simulink model "third"  (Simulink 7.2)
settings: Solver=ode15s  StartTime=0.0  StopTime=.6  RelTol=1e-3
libraries: powerlib x22, powerlib_extras x13
settings Model: Creator=User  LastModifiedBy=hamed
settings DataIOCC: SaveFormat=StructureWithTime

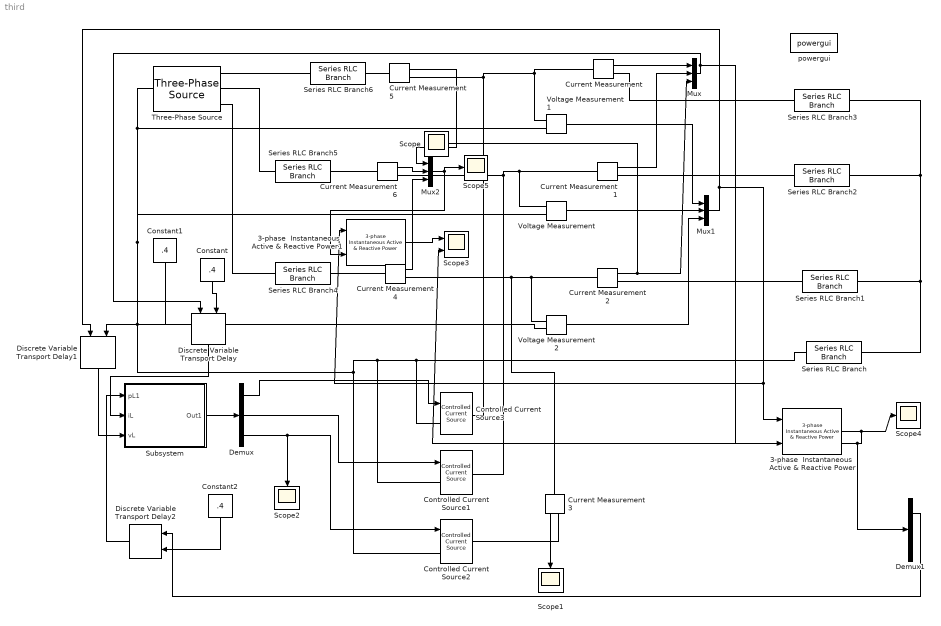
== system third ==
  3-phase  Instantaneous  Active & Reactive Power : powerlib_extras/Measurements/3-phase  Instantaneous  Active & Reactive Power  DialogController=POWERSYS.PowerSysDialog  SystemSampleTime=-1
  3-phase  Instantaneous  Active & Reactive Power1 : powerlib_extras/Measurements/3-phase  Instantaneous  Active & Reactive Power  DialogController=POWERSYS.PowerSysDialog  SystemSampleTime=-1
  Constant : Constant  Orientation=down  Value=.4  OutDataType=sfix(16)  OutScaling=2^0
  Constant1 : Constant  Orientation=down  Value=.4  OutDataType=sfix(16)  OutScaling=2^0
  Constant2 : Constant  Orientation=down  Value=.4  OutDataType=sfix(16)  OutScaling=2^0
  Controlled Current Source1 : powerlib/Electrical Sources/Controlled Current Source  DialogController=POWERSYS.PowerSysDialog  SystemSampleTime=-1  Initialize=on  Source_Type=AC  Amplitude=0  Phase=0  Frequency=0  Measurements=None
  Controlled Current Source2 : powerlib/Electrical Sources/Controlled Current Source  DialogController=POWERSYS.PowerSysDialog  SystemSampleTime=-1  Initialize=on  Source_Type=AC  Amplitude=0  Phase=0  Frequency=0  Measurements=None
  Controlled Current Source3 : powerlib/Electrical Sources/Controlled Current Source  DialogController=POWERSYS.PowerSysDialog  SystemSampleTime=-1  Initialize=on  Source_Type=AC  Amplitude=0  Phase=0  Frequency=0  Measurements=None
  Current Measurement{,1..2,4..6} (6 alike) : powerlib/Measurements/Current Measurement  DialogController=POWERSYS.PowerSysDialog  SystemSampleTime=-1  PhasorSimulation=off  OutputType=Complex  PSBequivalent=0
  Current Measurement3 : powerlib/Measurements/Current Measurement  Orientation=down  DialogController=POWERSYS.PowerSysDialog  SystemSampleTime=-1  PhasorSimulation=off  OutputType=Complex  PSBequivalent=0
  Demux : Demux  Outputs=3
  Demux1 : Demux  Outputs=2
  Discrete Variable Transport Delay : powerlib_extras/Discrete  Control Blocks/Discrete Variable Transport Delay  Orientation=down  DialogController=POWERSYS.PowerSysDialog  SystemSampleTime=-1  MaxDelay=1/40  InitialValue=0  Ts=50e-6
  Discrete Variable Transport Delay1 : powerlib_extras/Discrete  Control Blocks/Discrete Variable Transport Delay  Orientation=down  DialogController=POWERSYS.PowerSysDialog  SystemSampleTime=-1  MaxDelay=1/40  InitialValue=0  Ts=50e-6
  Discrete Variable Transport Delay2 : powerlib_extras/Discrete  Control Blocks/Discrete Variable Transport Delay  Orientation=left  DialogController=POWERSYS.PowerSysDialog  SystemSampleTime=-1  MaxDelay=1/40  InitialValue=0  Ts=50e-6
  Mux : Mux  Inputs=3
  Mux1 : Mux  Inputs=3
  Mux2 : Mux  Inputs=3
  Scope{,1..2,4..5} (5 alike) : Scope
      Scope settings: TimeRange=2  YMin=-125  YMax=200  SaveName=ScopeData2
      Scope1 settings: Orientation=down  TimeRange=2  YMin=-1000  YMax=1000  SaveName=ScopeData3
      Scope2 settings: Orientation=down  TimeRange=0.5  YMin=-100  YMax=200  SaveName=ScopeData4
      Scope4 settings: TimeRange=0.25  YMin=0  YMax=42500  SaveName=ScopeData8
      Scope5 settings: TimeRange=0.6  YMin=-1100  YMax=1000  SaveName=ScopeData5
  Scope3 : Scope  NumInputPorts=2
      settings: TimeRange=0.1  YMin=-5000~-20000  YMax=20000~40000  SaveName=ScopeData6
  Series RLC Branch{,4..6} (4 alike) : powerlib/Elements/Series RLC Branch  DialogController=POWERSYS.PowerSysDialog  PhysicalDomain=powersysdomain  SubClassName=unknown  LeftPortType=p1  RightPortType=p1  LConnTagsString=__new0  RConnTagsString=__new0  BranchType=R  Resistance=1  Inductance=1.0  SetiL0=off  InitialCurrent=0  Capacitance=1.0  Setx0=off  InitialVoltage=0  Measurements=None
  Series RLC Branch1 : powerlib/Elements/Series RLC Branch  DialogController=POWERSYS.PowerSysDialog  PhysicalDomain=powersysdomain  SubClassName=unknown  LeftPortType=p1  RightPortType=p1  LConnTagsString=__new0  RConnTagsString=__new0  BranchType=R  Resistance=1.0  Inductance=1.0  SetiL0=off  InitialCurrent=0  Capacitance=1.0  Setx0=off  InitialVoltage=0  Measurements=None
  Series RLC Branch2 : powerlib/Elements/Series RLC Branch  DialogController=POWERSYS.PowerSysDialog  PhysicalDomain=powersysdomain  SubClassName=unknown  LeftPortType=p1  RightPortType=p1  LConnTagsString=__new0  RConnTagsString=__new0  BranchType=R  Resistance=40  Inductance=1.0  SetiL0=off  InitialCurrent=0  Capacitance=1.0  Setx0=off  InitialVoltage=0  Measurements=None
  Series RLC Branch3 : powerlib/Elements/Series RLC Branch  DialogController=POWERSYS.PowerSysDialog  PhysicalDomain=powersysdomain  SubClassName=unknown  LeftPortType=p1  RightPortType=p1  LConnTagsString=__new0  RConnTagsString=__new0  BranchType=R  Resistance=100  Inductance=1.0  SetiL0=off  InitialCurrent=0  Capacitance=1.0  Setx0=off  InitialVoltage=0  Measurements=None
  Subsystem : Subsystem
  Three-Phase Source : powerlib/Electrical Sources/Three-Phase Source  DialogController=POWERSYS.PowerSysDialog  SystemSampleTime=-1  Voltage=380  PhaseAngle=0  Frequency=50  InternalConnection=Yn  SpecifyImpedance=on  Resistance=0.8929  Inductance=16.58e-3  ShortCircuitLevel=100e6  BaseVoltage=380  XRratio=7
  Voltage Measurement : powerlib/Measurements/Voltage Measurement  DialogController=POWERSYS.PowerSysDialog  SystemSampleTime=-1  PhasorSimulation=off  OutputType=Complex  PSBequivalent=0
  Voltage Measurement1 : powerlib/Measurements/Voltage Measurement  DialogController=POWERSYS.PowerSysDialog  SystemSampleTime=-1  PhasorSimulation=off  OutputType=Complex  PSBequivalent=0
  Voltage Measurement2 : powerlib/Measurements/Voltage Measurement  DialogController=POWERSYS.PowerSysDialog  SystemSampleTime=-1  PhasorSimulation=off  OutputType=Complex  PSBequivalent=0
  powergui : powerlib/powergui  SystemSampleTime=-1  SimulationMode=Continuous  SampleTime=50e-6  frequency=60  SPID=off  DisableSnubberDevices=off  DisableRonSwitches=off  DisableVfSwitches=off  SwTol=0  Interpol=off  frequencyindice=0  echomessages=off  HookPort=off  FunctionMessages=off  EnableUseOfTLC=off  x0status=blocks  RestoreLinks=warning  Frange=[0:2:500]  Ylog=off  Xlog=on  ShowGrid=off  save=off  variable=ZData  ZoomFFT=on  StartTime=0.0  cycles=1  DisplayStyle=1  fundamental=60  FreqAxis=off  MaxFrequency=1000  frequencyindicesteady=1  RmsSteady=1  display=off  Ts=0  methode=off
  wires:
  Current Measurement1/1 -> Mux/2
  Current Measurement2/1 -> Mux/3, Scope/1
  Voltage Measurement/1 -> Mux1/2
  Voltage Measurement2/1 -> Mux1/3
  Voltage Measurement1/1 -> Mux1/1
  Demux/1 -> Controlled Current Source3/1
  Demux/2 -> Controlled Current Source1/1
  Demux/3 -> Controlled Current Source2/1, Scope2/1
  Current Measurement3/1 -> Scope1/1
  Current Measurement/1 -> Mux/1
  Mux/1 -> Discrete Variable Transport Delay/1, 3-phase  Instantaneous  Active & Reactive Power/2
  Constant/1 -> Discrete Variable Transport Delay/2
  Mux1/1 -> Discrete Variable Transport Delay1/1, 3-phase  Instantaneous  Active & Reactive Power/1, 3-phase  Instantaneous  Active & Reactive Power1/1
  Constant1/1 -> Discrete Variable Transport Delay1/2
  3-phase  Instantaneous  Active & Reactive Power/1 -> Scope4/1, Scope3/2, Demux1/1
  Current Measurement5/1 -> Mux2/1
  Current Measurement6/1 -> Mux2/2
  Current Measurement4/1 -> Mux2/3
  3-phase  Instantaneous  Active & Reactive Power1/1 -> Scope3/1
  Mux2/1 -> 3-phase  Instantaneous  Active & Reactive Power1/2, Scope5/1
  Demux1/1 -> Discrete Variable Transport Delay2/1
  Constant2/1 -> Discrete Variable Transport Delay2/2
  Discrete Variable Transport Delay2/1 -> Subsystem/1(pL1)
  Discrete Variable Transport Delay/1 -> Subsystem/2(iL)
  Discrete Variable Transport Delay1/1 -> Subsystem/3(vL)
  Subsystem/1(Out1) -> Demux/1
  connections:
  Controlled Current Source3/RConn1 -- Current Measurement/LConn1 -- Voltage Measurement1/LConn1 -- Current Measurement5/RConn1
  Series RLC Branch/LConn1 -- Controlled Current Source3/LConn1 -- Controlled Current Source1/LConn1 -- Voltage Measurement/LConn2 -- Three-Phase Source/LConn1 -- Voltage Measurement1/LConn2 -- Voltage Measurement2/LConn2 -- Controlled Current Source2/LConn1
  Current Measurement3/LConn1 -- Current Measurement2/LConn1 -- Voltage Measurement2/LConn1 -- Current Measurement4/RConn1
  Current Measurement1/RConn1 -- Series RLC Branch2/LConn1
  Current Measurement2/RConn1 -- Series RLC Branch1/LConn1
  Series RLC Branch3/RConn1 -- Series RLC Branch/RConn1 -- Series RLC Branch1/RConn1 -- Series RLC Branch2/RConn1
  Current Measurement/RConn1 -- Series RLC Branch3/LConn1
  Series RLC Branch6/LConn1 -- Three-Phase Source/RConn1
  Three-Phase Source/RConn2 -- Series RLC Branch5/LConn1
  Three-Phase Source/RConn3 -- Series RLC Branch4/LConn1
  Controlled Current Source2/RConn1 -- Current Measurement3/RConn1
  Current Measurement4/LConn1 -- Series RLC Branch4/RConn1
  Current Measurement5/LConn1 -- Series RLC Branch6/RConn1
  Current Measurement6/LConn1 -- Series RLC Branch5/RConn1
  Controlled Current Source1/RConn1 -- Current Measurement1/LConn1 -- Voltage Measurement/LConn1 -- Current Measurement6/RConn1

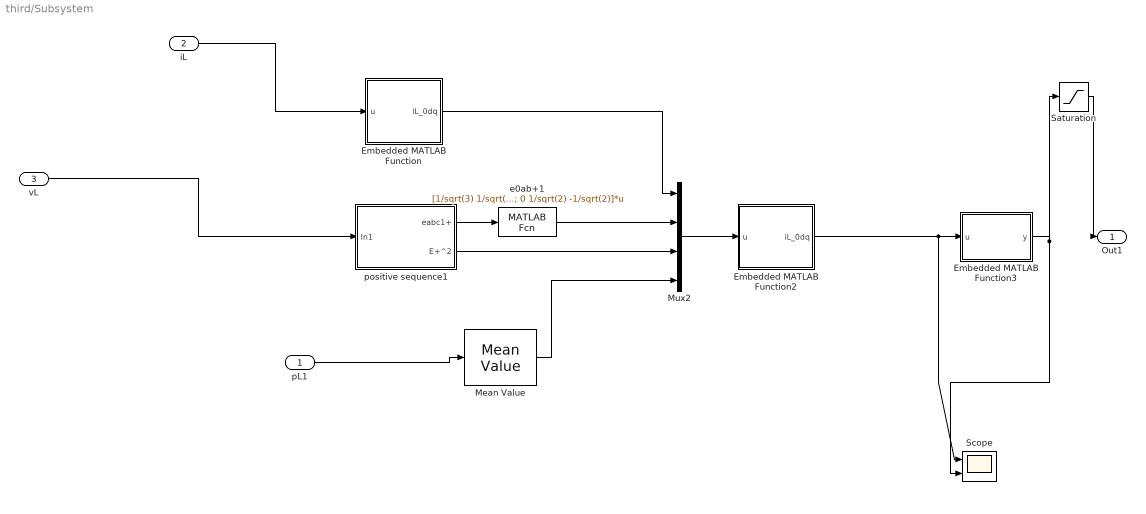
== system third/Subsystem ==
  pL1 : Inport  OutDataType=fixdt(1, 16)  OutScaling=2^0
  iL : Inport  Port=2  OutDataType=fixdt(1, 16)  OutScaling=2^0
  vL : Inport  Port=3  OutDataType=fixdt(1, 16)  OutScaling=2^0
  Embedded MATLAB Function : Stateflow chart  TreatAsAtomicUnit=on
  Embedded MATLAB Function2 : Stateflow chart  TreatAsAtomicUnit=on
  Embedded MATLAB Function3 : Stateflow chart  TreatAsAtomicUnit=on
  Mean Value : powerlib_extras/Measurements/Mean Value  DialogController=POWERSYS.PowerSysDialog  SystemSampleTime=-1  Period=1/60
  Mux2 : Mux
  Saturation : Saturate  UpperLimit=1000  LowerLimit=-1000  OutDataType=sfix(16)  OutScaling=2^0
  Scope : Scope  NumInputPorts=2
      settings: YMin=-250~-200  YMax=250~200
  e0ab+1 : MATLABFcn  MATLABFcn=[1/sqrt(3) 1/sqrt(3) 1/sqrt(3); sqrt(2)/sqrt(3) -1/sqrt(6) -1/sqrt(6); 0 1/sqrt(2) -1/sqrt(2)]*u
  positive sequence1 : Subsystem
  Out1 : Outport  OutDataType=fixdt(1, 16)  OutScaling=2^0
  wires:
  pL1/1 -> Mean Value/1
  Embedded MATLAB Function/1(iL_0dq) -> Mux2/1
  e0ab+1/1 -> Mux2/2
  Mean Value/1 -> Mux2/4
  Mux2/1 -> Embedded MATLAB Function2/1(u)
  Embedded MATLAB Function2/1(iL_0dq) -> Scope/1, Embedded MATLAB Function3/1(u)
  Embedded MATLAB Function3/1(y) -> Scope/2, Saturation/1
  positive sequence1/2(E+^2) -> Mux2/3
  positive sequence1/1(eabc1+) -> e0ab+1/1
  Saturation/1 -> Out1/1
  iL/1 -> Embedded MATLAB Function/1(u)
  vL/1 -> positive sequence1/1(In1)

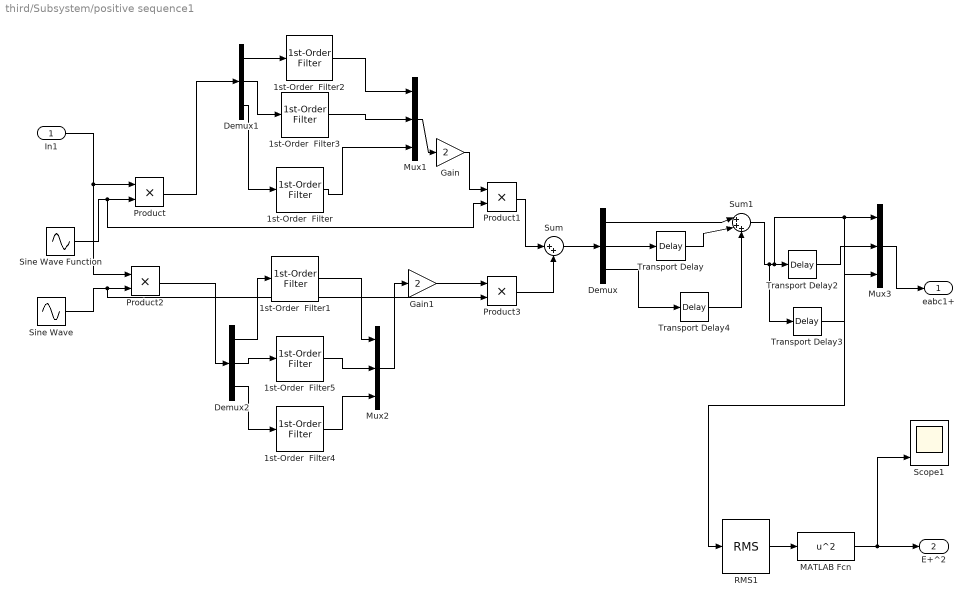
== system third/Subsystem/positive sequence1 ==
  In1 : Inport  OutDataType=sfix(16)  OutScaling=2^0
  1st-Order  Filter{,1..5} (6 alike) : powerlib_extras/Control  Blocks/1st-Order  Filter  DialogController=POWERSYS.PowerSysDialog  SystemSampleTime=-1  FilterType=Lowpass  Tc=.01  Initialize=off  Vac_Init=[0.8 -25 60]  Vdc_Init=-0.4  PlotResponse=off  param1=[1 500 1]
  Demux : Demux  Outputs=3
  Demux1 : Demux  Outputs=3
  Demux2 : Demux  Outputs=3
  Gain : Gain  Gain=2  ParameterDataType=sfix(16)  ParameterScaling=2^0  OutDataType=sfix(16)  OutScaling=2^0
  Gain1 : Gain  Gain=2  ParameterDataType=sfix(16)  ParameterScaling=2^0  OutDataType=sfix(16)  OutScaling=2^0
  MATLAB Fcn : MATLABFcn  MATLABFcn=u^2
  Mux1 : Mux  Inputs=3
  Mux2 : Mux  Inputs=3
  Mux3 : Mux  Inputs=3
  Product{,1..3} (4 alike) : Product  OutDataType=sfix(16)  OutScaling=2^0  RndMeth=Zero
  RMS1 : powerlib_extras/Measurements/RMS  DialogController=POWERSYS.PowerSysDialog  SystemSampleTime=-1  f1=50
  Scope1 : Scope  NumInputPorts=3
      settings: YMin=-1~-1~150000  YMax=1~1~320000
  Sine Wave : Sin  Frequency=100*pi  Phase=pi/2  SampleTime=0
  Sine Wave Function : Sin  Frequency=100*pi  SampleTime=0
  Sum : Sum  Inputs=|++  OutDataType=sfix(16)  OutScaling=2^0
  Sum1 : Sum  Inputs=|+++  OutDataType=sfix(16)  OutScaling=2^0
  Transport Delay : TransportDelay  DelayTime=.04/3
  Transport Delay2 : TransportDelay  DelayTime=.02/3
  Transport Delay3 : TransportDelay  DelayTime=.04/3
  Transport Delay4 : TransportDelay  DelayTime=.02/3
  eabc1+ : Outport  OutDataType=sfix(16)  OutScaling=2^0
  E+^2 : Outport  Port=2  OutDataType=sfix(16)  OutScaling=2^0
  wires:
  RMS1/1 -> MATLAB Fcn/1
  MATLAB Fcn/1 -> E+^2/1, Scope1/3
  In1/1 -> Product/1, Product2/1
  Sine Wave Function/1 -> Product/2, Product1/2
  1st-Order  Filter/1 -> Mux1/3
  Gain/1 -> Product1/1
  Sine Wave/1 -> Product2/2, Product3/2
  Gain1/1 -> Product3/1
  Product1/1 -> Sum/1
  Product3/1 -> Sum/2
  Sum/1 -> Demux/1
  Demux/2 -> Transport Delay/1
  Demux/1 -> Sum1/1
  Transport Delay/1 -> Sum1/2
  Sum1/1 -> Transport Delay3/1, Transport Delay2/1, Mux3/1, RMS1/1
  Transport Delay4/1 -> Sum1/3
  Demux/3 -> Transport Delay4/1
  Transport Delay2/1 -> Mux3/2
  Transport Delay3/1 -> Mux3/3
  Mux3/1 -> eabc1+/1
  Demux1/1 -> 1st-Order  Filter2/1
  Demux1/2 -> 1st-Order  Filter3/1
  Demux1/3 -> 1st-Order  Filter/1
  Product/1 -> Demux1/1
  Demux2/1 -> 1st-Order  Filter1/1
  Demux2/2 -> 1st-Order  Filter5/1
  Demux2/3 -> 1st-Order  Filter4/1
  Product2/1 -> Demux2/1
  1st-Order  Filter2/1 -> Mux1/1
  1st-Order  Filter3/1 -> Mux1/2
  Mux1/1 -> Gain/1
  1st-Order  Filter1/1 -> Mux2/1
  1st-Order  Filter5/1 -> Mux2/2
  1st-Order  Filter4/1 -> Mux2/3
  Mux2/1 -> Gain1/1

== matlab function Subsystem/Embedded MATLAB Function ==
  data: u input double; iL_0dq output double
function iL_0dq = fcn(u)
%#eml

iL_0dq =[1/sqrt(3) 1/sqrt(3) 1/sqrt(3); sqrt(2)/sqrt(3) -sqrt(2)/(2*sqrt(3)) -sqrt(2)/(2*sqrt(3)); 0 1/sqrt(2) -1/sqrt(2)]*u;

== matlab function Subsystem/Embedded MATLAB Function2 ==
  data: u input double; iL_0dq output double
function iL_0dq = fcn(u)
%#eml
if u(7)==0
    iL_0dq=[0;0;0];
else
iL_0dq =[u(1);u(2);u(3)]-(u(8)/u(7))*[0;u(5);u(6)];
end

== matlab function Subsystem/Embedded MATLAB Function3 ==
  data: u input double; y output double
function y = fcn(u)
%#eml

y =[1/sqrt(3) sqrt(2)/sqrt(3) 0 ;1/sqrt(3) -sqrt(2)/(2*sqrt(3)) 1/sqrt(2) ;1/sqrt(3) -sqrt(2)/(2*sqrt(3)) -1/sqrt(2)]*u;
